simulink model "SVPWM_nosense"  (R2023b)
settings: Solver=FixedStepAuto  StartTime=0.0  StopTime=50  FixedStep=5e-7  RelTol=1e-3
libraries: slpidlib x10, dspfdesign x7, spsMosfetLib x6, mcbcontrolslib x4, simulink x3, spsDCVoltageSourceLib x1, spsPermanentMagnetSynchronousMachineLib x1, sps_lib x1, spsSVPWMGenerator2LevelLib x1, spsSawtoothGeneratorLib x1
(part 2 of 2)

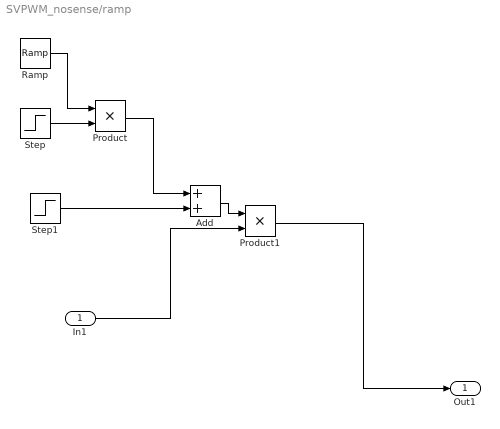
== system SVPWM_nosense/ramp ==
  In1 : Inport
  Add : Sum
  Product : Product
  Product1 : Product
  Ramp : simulink/Sources/Ramp  slope=0.2  start=0  InitialOutput=0.2
  Step : Step  Time=4  Before=1  After=0  SampleTime=0
  Step1 : Step  Time=4  SampleTime=0
  Out1 : Outport
  wires:
  Step/1 -> Product/2
  Add/1 -> Product1/1
  Product/1 -> Add/1
  In1/1 -> Product1/2
  Step1/1 -> Add/2
  Ramp/1 -> Product/1
  Product1/1 -> Out1/1

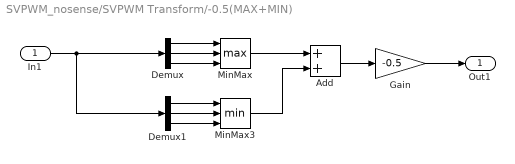
== system SVPWM_nosense/SVPWM Transform/-0.5(MAX+MIN) ==
  In1 : Inport
  Add : Sum
  Demux : Demux  Outputs=3
  Demux1 : Demux  Outputs=3
  Gain : Gain  Gain=-0.5
  MinMax : MinMax  Function=max  Inputs=3
  MinMax3 : MinMax  Inputs=3
  Out1 : Outport
  wires:
  In1/1 -> Demux1/1, Demux/1
  Demux/1 -> MinMax/1
  Demux/2 -> MinMax/2
  Demux/3 -> MinMax/3
  Demux1/1 -> MinMax3/1
  Demux1/2 -> MinMax3/2
  Demux1/3 -> MinMax3/3
  MinMax/1 -> Add/1
  MinMax3/1 -> Add/2
  Add/1 -> Gain/1
  Gain/1 -> Out1/1

== matlab function SVPWM_nosense/MATLAB Function1 ==
  settings: updateMethod=DISCRETE  sampleTime=0.000005
  data: x input; v_prime output; Omega input; k input; qv_prime output
function [v_prime, qv_prime] = SOGI_Dynamic(x, Omega, k)
% 输入：
%   x: 输入信号
%   Omega: 中心频率（rad/s）
%   k: 阻尼系数（固定参数，可封装为模块参数）
% 输出：
%   v_prime: 同相输出
%   qv_prime: 正交输出

% 持久化变量（状态量）
persistent x1 x2
if isempty(x1)
    x1 = 0; % 初始状态 x1
    x2 = 0; % 初始状态 x2
end

% 连续状态方程（离散化采用前向欧拉法，需定义采样时间 Ts）
Ts = 0.000005; % 示例采样时间，需与实际模型一致

% 状态更新
dx1 = x2;
dx2 = -k*Omega*x2 - Omega^2*x1 + k*Omega*x;

% 离散化（欧拉法）
x1 = x1 + dx1 * Ts;
x2 = x2 + dx2 * Ts;

% 输出
v_prime = x2;
qv_prime = Omega * x1;
end
